simulink model "VirtualOscilloscope_stable"  (R2021b)
settings: Solver=VariableStepAuto  StartTime=0.0  StopTime=inf  MaxStep=0.001  RelTol=1e-3
PostLoadFcn:
  | % Resize the model window
  | set(0,"Units","pixels")
  | sSize = get(0,"screensize");
  | space =  sSize(4)*0.028;
  | set_param(gcs,'location',  [1,1,round(sSize(3)/2),sSize(4)-space]);
  | % Reset the zoom
  | set_param(gcs, 'ZoomFactor','FitSystem')
  | 
  | % Resize the windows
  | space = sSize(4)*0.032;
  | SAsize = ['[',num2str(round([(sSize(3)/2)+1,...
  |                     space,(sSize(3)/2)-1,sSize(4)/2-space*1.25])),']'];
  | DSOsize = ['[',num2str(round([(sSize(3)/2)+1,...
  |                   space/2+sSize(4)/2,(sSize(3)/2)-1,sSize(4)/2-1.25*space])),']'];
  | set_param([gcs,'/Signal Analyzer'],'WindowPosition',SAsize)
  | set_param([gcs,'/Oscilloscope'],'WindowPosition',DSOsize)
libraries: fl_lib x5, nesl_utility x3, simulink x2, ee_lib x1, dspxfrm3 x1
(part 1 of 2)
settings Model: Creator=Work  LastModifiedBy=Work

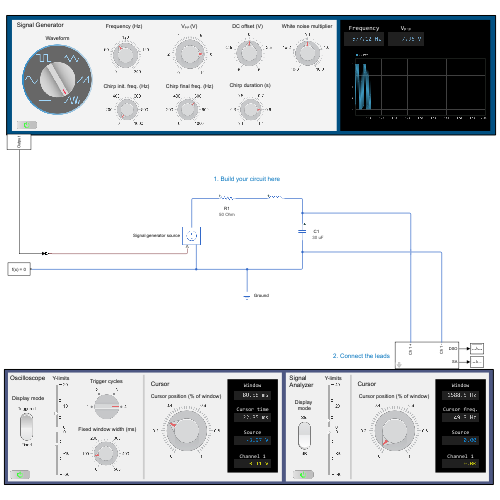
[thumbnail: Simulink's stored preview of the top-level diagram]
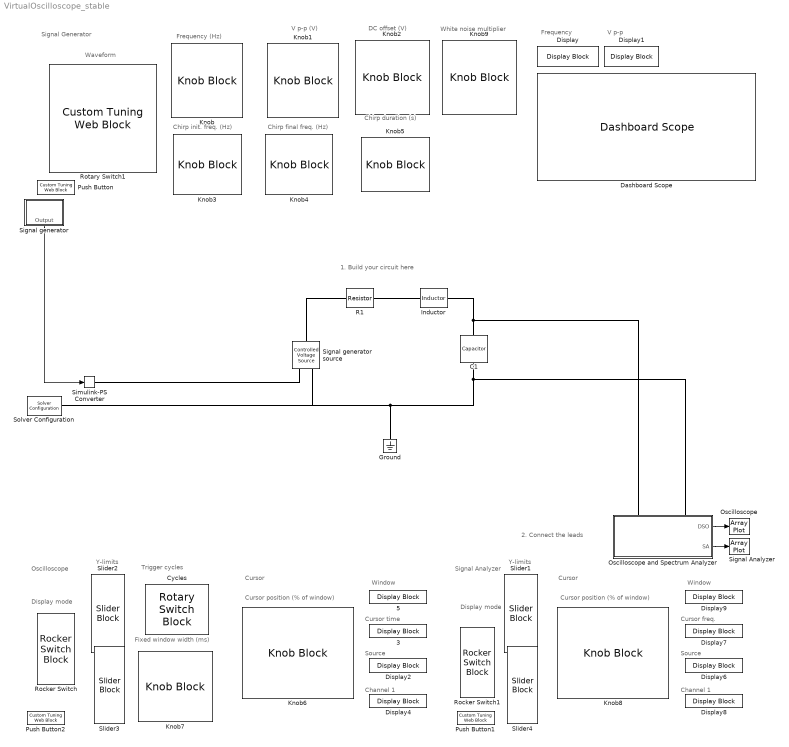
== system VirtualOscilloscope_stable ==
  note: 1. Build your circuit here
  note: Frequency (Hz)
  note: Waveform
  note: V p-p (V)
  note: Signal Generator
  note: Trigger cycles
  note: DC offset (V)
  note: Frequency
  note: V p-p
  note: Chirp init. freq. (Hz)
  note: Chirp final freq. (Hz)
  note: Source
  note: 2. Connect the leads
  note: Cursor position (% of window)
  note: Channel 1
  note: Cursor time
  note: Display mode
  note: Fixed window width (ms)
  note: Oscilloscope
  note: Window
  note: Cursor
  note: Window
  note: Cursor
  note: Channel 1
  note: Cursor position (% of window)
  note: Source
  note: Cursor freq.
  note: Chirp duration (s)
  note: Y-limits
  note: Display
      | mode
  note: Y-limits
  note: White noise multiplier
  note: Signal
      | Analyzer
  3 : DisplayBlock  LabelPosition=Hide  Format=Custom  Alignment=Right  Transparency=1  FormatString=%0.2f ms
  5 : DisplayBlock  LabelPosition=Hide  Format=Custom  Alignment=Right  Transparency=1  FormatString=%0.2f ms
  C1 : fl_lib/Electrical/Electrical Elements/Capacitor  c=30 uF  r=1e-6 Ohm  g=0 1/Ohm  i_specify=off  i_priority=None  i=0 A  i_nominal_specify=off  i_nominal_unit=A  i_nominal_value=1  v_specify=off  v_priority=None  v=0 V  v_nominal_specify=off  v_nominal_unit=V  v_nominal_value=1  vc_specify=off  vc_priority=High  vc=0 V  vc_nominal_specify=off  vc_nominal_unit=V  vc_nominal_value=1
      settings: AttributesFormatString=%<c> %<c_unit>
  Cycles : RotarySwitchBlock  LabelPosition=Hide
      settings: Values={{'1', '2', '3', '4'}, [1 2 3 4]}
  Dashboard Scope : DashboardScope  TimeSpan=0.20000000000000001  Ymin=-5  Ymax=5  ScaleAtStop=off
  Display : DisplayBlock  LabelPosition=Hide  Format=Custom  Alignment=Right  Transparency=1  FormatString=%0.2f Hz
  Display1 : DisplayBlock  LabelPosition=Hide  Format=Custom  Alignment=Right  Transparency=1  FormatString=%0.2f V
  Display2 : DisplayBlock  LabelPosition=Hide  Format=Custom  Alignment=Right  Transparency=1  FormatString=%0.2f V
  Display4 : DisplayBlock  LabelPosition=Hide  Format=Custom  Alignment=Right  Transparency=1  FormatString=%0.2f V
  Display6 : DisplayBlock  LabelPosition=Hide  Format=Custom  Alignment=Right  Transparency=1  FormatString=%0.2f
  Display7 : DisplayBlock  LabelPosition=Hide  Format=Custom  Alignment=Right  Transparency=1  FormatString=%0.1f Hz
  Display8 : DisplayBlock  LabelPosition=Hide  Format=Custom  Alignment=Right  Transparency=1  FormatString=%0.2f
  Display9 : DisplayBlock  LabelPosition=Hide  Format=Custom  Alignment=Right  Transparency=1  FormatString=%0.1f Hz
  Ground : fl_lib/Electrical/Electrical Elements/Electrical Reference
  Inductor : ee_lib/Passive/Inductor  l=0.1 H  L_tol=20  enable_L_tol=0  tol_distribution=1  nSigma=4  r=0 Ohm  g=1e-9 1/Ohm  enable_operating_limits=0  operating_limit_action=2  max_working_current=1 A  power_rating=1 W  enable_faults=0  fault_action=1  lambdaPercent=50  k_faulted=0.9999  turnsShort=0  openCct=0  groundShort=0  groundShortG=0 1/Ohm  tau_fault=1e-3 s  enable_temporal_fault=0  t_fault=1 s  enable_behavioral_fault=0  max_permissible_voltage=100 V  n_fail_on_voltage=1  max_permissible_current=1 A  t_fail_on_current=1 s  i_L_specify=off  i_L_priority=High  i_L=0 A  i_L_nominal_specify=off  i_L_nominal_unit=A  i_L_nominal_value=1
  Knob : KnobBlock  LabelPosition=Hide  ScaleMax=240  TickInterval=60
  Knob1 : KnobBlock  LabelPosition=Hide  ScaleMax=10  TickInterval=2
  Knob2 : KnobBlock  LabelPosition=Hide  ScaleMin=-5  ScaleMax=5  TickInterval=2.5
  Knob3 : KnobBlock  LabelPosition=Hide  ScaleMax=1000  TickInterval=200
  Knob4 : KnobBlock  LabelPosition=Hide  ScaleMax=1000  TickInterval=200
  Knob5 : KnobBlock  LabelPosition=Hide  ScaleMin=0.1  ScaleMax=1.1  TickInterval=0.2
  Knob6 : KnobBlock  LabelPosition=Hide  ScaleMax=1  TickInterval=0.2
  Knob7 : KnobBlock  LabelPosition=Hide  ScaleMax=500  TickInterval=100
  Knob8 : KnobBlock  LabelPosition=Hide  ScaleMax=1  TickInterval=0.2
  Knob9 : KnobBlock  LabelPosition=Hide  ScaleMin=1e-3  ScaleMax=10  ScaleType=Log
  Oscilloscope : ArrayPlot  WindowPosition=[1281.000000,743.000000,1279.000000,662.000000,]  Visible=on  PlotType=Line  AxesScaling=Manual  MaximizeAxes=off  YLimits=[-5.751633986928104,6.405228758169934]  ShowLegend=on
  Oscilloscope and Spectrum Analyzer : Subsystem  mask{Np=256, plot_dt=0.5e-5, refreshRate=100}
      mask prompts: Np "Sample points"; plot_dt "Sample time (s)"; refreshRate "Plot refresh rate (Hz)"
      settings: PortSchema="{\"entries\":[{\"content\":{\"sides\":[{\"content\":{\"connectorIds\":[\"LConn1\",\"LConn2\"]},\"type\":\"ConnectorPlacement.EquallySpacedRectSide\",\"uuid\":\"4f80a8c2-824d-4211-993f-82229c097a2c\"},{\"content\":{\"connectorIds\":[],\"side\":\"RIGHT\"},\"type\":\"ConnectorPlacement.EquallySpacedRectSide\",\"uuid\":\"5753fbaa-289b-4ec3-ae4c-c42164e19fcd\"},{\"content\":{\"connectorIds\":[\"Out1\",\"Out2\"],\"side\":\"TOP\"},\"type\":\"ConnectorPlacement.EquallySpacedRectSide\",\"uuid\":\"cde524b8-672e-4186-b31f-d28de61f9925\"}]},\"type\":\"ConnectorPlacement.EquallySpacedConnector\",\"uuid\":\"ab826d68-b3e0-4882-8d23-163848ab4439\"}],\"packageUris\":[\"http://schema.mathworks.com/mf0/Connector/R2020b\"],\"version\":\"1.0\"}"
  Push Button : CustomTuningWebBlock  LabelPosition=Hide  ShowInitialText=on  Configuration="{\"components\":[{\"name\":\"BackgroundImageComponent\",\"settings\":{\"image\":{\"size\":[0,0],\"src\":\"default\",\"srcOrientation\":\"horizontal\"},\"position\":[0,0,1,1],\"scaleMode\":\"0\"}},{\"name\":\"ButtonStateComponent\",\"settings\":{\"buttonType\":\"latch\",\"clickFcn\":\"\",\"latched\":true,\"offValue\":0,\"onValue\":1,\"position\":[0,0,1,1],\"pressDelay\":500,\"pressFcn\":\"\",\"repeatInterval\":0,\"states\":[{\"horizontalAlignment\":\"center\",\"image\":{\"position\":[0,0.07949909875723365,0.8410018024855327,1],\"size\":[0.8410018024855327,1],\"src\":\"data:image\\/png;base64,iVBORw0KGgoAAAANSUhEUgAAAk8AAAD+CAYAAAAjzuGXAAAACXBIWXMAAC4lAAAuJQH4pnvtAAAAGXRFWHRTb2Z0d2FyZQB3d3cuaW5rc2NhcGUub3Jnm+48GgAAIABJREFUeJzt3XlwHNmdH\\/jvyyqgTqCAKtwgSJDgfTXJNtmnRKK7R9LMyJJnvR7Je8xGeL3aXccqPLIVmlZPE85mt9QahRQay+GdjfGMZU9412PZO7cdY89oBTY9Gh3NJkV2N08QvAAQRxWAQhXqzrd\\/dAMiicxCHZmVWVXfTwRDYuXL937NArJ+9U4BeoSqqt5CoTAihBgGMCyEGBZC9EopI0KIiJQyAiAshBAA3FLKNlsDJiIiKpMQYgVAXkopAcSEEFEpZVQIEQXw ...(+19432 chars)\",\"srcOrientation\":\"Right\"},\"label\":{\"color\":[0.9176470588235294,0.9176470588235294,0.9176470588235294],\"icon\":{\"size\":[0,0],\"src\":\"default\",\"srcOrientation\":\"Right\"},\"iconPlacement\":\"left\",\"opacity\":1,\"show\":true,\"text\":{\"content\":\"\",\"font\":\"Helvetica\",\"fontSize\":42}},\"labelOffset\":[-0.019507668917408183,0.0018518518518518268],\"verticalAlignment\":\"middle\"},{\"horizontalAlignment\":\"center\",\"image\":{\"position\":[0,0.07949909875723365,0.8410018024855327,1],\"size\":[0.8410018024855327,1],\"src\":\"data:image\\/png;base64,iVBORw0KGgoAAAANSUhEUgAAAk8AAAD+CAYAAAAjzuGXAAAACXBIWXMAAC4lAAAuJQH4pnvtAAAAGXRFWHRTb2Z0d2FyZQB3d3cuaW5rc2NhcGUub3Jnm+48GgAAIABJREFUeJzt3Xl4HMd5J\\/5v9Qzmxn0SIAnwpkhLJCVRkkUdACVb8hErjje2c2zy28RxsnniTZx4bVkRuS1Kthw\\/9uPEOZx1fCTOL5eTOL5vWaBoS1F0ixIpkQQB3gCIe2Ywd9f+QQIEMN0z3T3dMwPi+9Ejm+h+u6pIipiXVW9XCdAiqqoGcrncBiFED4AeIUSPEKJdStkshGiWUjYDaBJCCABeKWVtRQdMRERkkRAiCiArpZQAJoQQ41LKcSHEOIBhAEML\\/j2pqm ...(+24250 chars)\",\"srcOrientation\":\"Right\"},\"label\":{\"color\":[0.9176470588235294,0.9176470588235294,0.9176470588235294],\"icon\":{\"size\":[0,0],\"src\":\"default\",\"srcOrientation\":\"Right\"},\"iconPlacement\":\"top\",\"opacity\":1,\"show\":true,\"text\":{\"content\":\"\",\"font\":\"Helvetica\",\"fontSize\":42}},\"labelOffset\":[-0.017384370015948947,0.002777777777777768],\"verticalAlignment\":\"middle\"},{\"horizontalAlignment\":\"center\",\"image\":{\"position\":[0,0.07949909875723365,0.8410018024855327,1],\"size\":[0.8410018024855327,1],\"src\":\"data:image\\/png;base64,iVBORw0KGgoAAAANSUhEUgAAAk8AAAD+CAYAAAAjzuGXAAAACXBIWXMAAC4lAAAuJQH4pnvtAAAAGXRFWHRTb2Z0d2FyZQB3d3cuaW5rc2NhcGUub3Jnm+48GgAAIABJREFUeJzt3Xl4HMd5J\\/5v9Qzmxn0SIAnwpkhLJCVRkkUdACVb8hErjje2c2zy28RxsnniTZx4bVkRuS1Kthw\\/9uPEOZx1fCTOL5eTOL5vWaBoS1F0ixIpkQQB3gCIe2Ywd9f+QQIEMN0z3T3dMwPi+9Ejm+h+u6pIipiXVW9XCdAiqqoGcrncBiFED4AeIUSPEKJdStkshGiWUjYDaBJCCABeKWVtRQdMRERkkRAiCiArpZQAJoQQ41LKcSHEOIBhAEML\\/j2pqm ...(+24250 chars)\",\"srcOrientation\":\"Right\"},\"label\":{\"color\":[0.9176470588235294,0.9176470588235294,0.9176470588235294],\"icon\":{\"size\":[0,0],\"src\":\"default\",\"srcOrientation\":\"Right\"},\"iconPlacement\":\"left\",\"opacity\":1,\"show\":true,\"text\":{\"content\":\"\",\"font\":\"Helvetica\",\"fontSize\":21}},\"labelOffset\":[0,0],\"verticalAlignment\":\"middle\"},{\"horizontalAlignment\":\"center\",\"image\":{\"position\":[0,0.07949909875723365,0.8410018024855327,1],\"size\":[0.8410018024855327,1],\"src\":\"data:image\\/png;base64,iVBORw0KGgoAAAANSUhEUgAAAk8AAAD+CAYAAAAjzuGXAAAACXBIWXMAAC4lAAAuJQH4pnvtAAAAGXRFWHRTb2Z0d2FyZQB3d3cuaW5rc2NhcGUub3Jnm+48GgAAIABJREFUeJzt3Xl4HMd5J\\/5v9Qzmxn0SIAnwpkhLJCVRkkUdACVb8hErjje2c2zy28RxsnniTZx4bVkRuS1Kthw\\/9uPEOZx1fCTOL5eTOL5vWaBoS1F0ixIpkQQB3gCIe2Ywd9f+QQIEMN0z3T3dMwPi+9Ejm+h+u6pIipiXVW9XCdAiqqoGcrncBiFED4AeIUSPEKJdStkshGiWUjYDaBJCCABeKWVtRQdMRERkkRAiCiArpZQAJoQQ41LKcSHEOIBhAEML\\/j2pqm ...(+24250 chars)\",\"srcOrientation\":\"Right\"},\"label\":{\"color\":[0.9176470588235294,0.9176470588235294,0.9176470588235294],\"icon\":{\"size\":[0,0],\"src\":\"default\",\"srcOrientation\":\"Right\"},\"iconPlacement\":\"left\",\"opacity\":1,\"show\":true,\"text\":{\"content\":\"\",\"font\":\"Helvetica\",\"fontSize\":21}},\"labelOffset\":[0.025,0],\"verticalAlignment\":\"middle\"}]}},{\"name\":\"ForegroundImageComponent\",\"settings\":{\"image\":{\"size\":[0,0],\"src\":\"default\",\"srcOrientation\":\"horizontal\"},\"isForeground\":1,\"position\":[0,0,1,1],\"scaleMode\":\"0\"}}],\"settings\":{\"BindingType\":\"param\",\"aspectRatio\":3.7777777777777777,\"backgroundColor\":[0,0,0,\"1\"],\"backgroundOffset\":0,\"backgroundOpacity\":1,\"fixedAspectRatio\":\"on\",\"foregroundColor\":[252,252,196],\"showBackgroundColor\":false,\"variant\":\"push\"},\"type\":\"Button\"}"
  Push Button1 : CustomTuningWebBlock  LabelPosition=Hide  ShowInitialText=on  Configuration="{\"components\":[{\"name\":\"BackgroundImageComponent\",\"settings\":{\"image\":{\"size\":[0,0],\"src\":\"default\",\"srcOrientation\":\"horizontal\"},\"position\":[0,0,1,1],\"scaleMode\":\"0\"}},{\"name\":\"ButtonStateComponent\",\"settings\":{\"buttonType\":\"latch\",\"clickFcn\":\"\",\"latched\":true,\"offValue\":0,\"onValue\":1,\"position\":[0,0,1,1],\"pressDelay\":500,\"pressFcn\":\"\",\"repeatInterval\":0,\"states\":[{\"horizontalAlignment\":\"center\",\"image\":{\"position\":[0,0.07949909875723365,0.8410018024855327,1],\"size\":[0.8410018024855327,1],\"src\":\"data:image\\/png;base64,iVBORw0KGgoAAAANSUhEUgAAAk8AAAD+CAYAAAAjzuGXAAAACXBIWXMAAC4lAAAuJQH4pnvtAAAAGXRFWHRTb2Z0d2FyZQB3d3cuaW5rc2NhcGUub3Jnm+48GgAAIABJREFUeJzt3XlwHNmdH\\/jvyyqgTqCAKtwgSJDgfTXJNtmnRKK7R9LMyJJnvR7Je8xGeL3aXccqPLIVmlZPE85mt9QahRQay+GdjfGMZU9412PZO7cdY89oBTY9Gh3NJkV2N08QvAAQRxWAQhXqzrd\\/dAMiicxCHZmVWVXfTwRDYuXL937NArJ+9U4BeoSqqt5CoTAihBgGMCyEGBZC9EopI0KIiJQyAiAshBAA3FLKNlsDJiIiKpMQYgVAXkopAcSEEFEpZVQIEQXw ...(+19432 chars)\",\"srcOrientation\":\"Right\"},\"label\":{\"color\":[0.9176470588235294,0.9176470588235294,0.9176470588235294],\"icon\":{\"size\":[0,0],\"src\":\"default\",\"srcOrientation\":\"Right\"},\"iconPlacement\":\"left\",\"opacity\":1,\"show\":true,\"text\":{\"content\":\"\",\"font\":\"Helvetica\",\"fontSize\":42}},\"labelOffset\":[-0.019507668917408183,0.0018518518518518268],\"verticalAlignment\":\"middle\"},{\"horizontalAlignment\":\"center\",\"image\":{\"position\":[0,0.07949909875723365,0.8410018024855327,1],\"size\":[0.8410018024855327,1],\"src\":\"data:image\\/png;base64,iVBORw0KGgoAAAANSUhEUgAAAk8AAAD+CAYAAAAjzuGXAAAACXBIWXMAAC4lAAAuJQH4pnvtAAAAGXRFWHRTb2Z0d2FyZQB3d3cuaW5rc2NhcGUub3Jnm+48GgAAIABJREFUeJzt3Xl4HMd5J\\/5v9Qzmxn0SIAnwpkhLJCVRkkUdACVb8hErjje2c2zy28RxsnniTZx4bVkRuS1Kthw\\/9uPEOZx1fCTOL5eTOL5vWaBoS1F0ixIpkQQB3gCIe2Ywd9f+QQIEMN0z3T3dMwPi+9Ejm+h+u6pIipiXVW9XCdAiqqoGcrncBiFED4AeIUSPEKJdStkshGiWUjYDaBJCCABeKWVtRQdMRERkkRAiCiArpZQAJoQQ41LKcSHEOIBhAEML\\/j2pqm ...(+24250 chars)\",\"srcOrientation\":\"Right\"},\"label\":{\"color\":[0.9176470588235294,0.9176470588235294,0.9176470588235294],\"icon\":{\"size\":[0,0],\"src\":\"default\",\"srcOrientation\":\"Right\"},\"iconPlacement\":\"top\",\"opacity\":1,\"show\":true,\"text\":{\"content\":\"\",\"font\":\"Helvetica\",\"fontSize\":42}},\"labelOffset\":[-0.017384370015948947,0.002777777777777768],\"verticalAlignment\":\"middle\"},{\"horizontalAlignment\":\"center\",\"image\":{\"position\":[0,0.07949909875723365,0.8410018024855327,1],\"size\":[0.8410018024855327,1],\"src\":\"data:image\\/png;base64,iVBORw0KGgoAAAANSUhEUgAAAk8AAAD+CAYAAAAjzuGXAAAACXBIWXMAAC4lAAAuJQH4pnvtAAAAGXRFWHRTb2Z0d2FyZQB3d3cuaW5rc2NhcGUub3Jnm+48GgAAIABJREFUeJzt3Xl4HMd5J\\/5v9Qzmxn0SIAnwpkhLJCVRkkUdACVb8hErjje2c2zy28RxsnniTZx4bVkRuS1Kthw\\/9uPEOZx1fCTOL5eTOL5vWaBoS1F0ixIpkQQB3gCIe2Ywd9f+QQIEMN0z3T3dMwPi+9Ejm+h+u6pIipiXVW9XCdAiqqoGcrncBiFED4AeIUSPEKJdStkshGiWUjYDaBJCCABeKWVtRQdMRERkkRAiCiArpZQAJoQQ41LKcSHEOIBhAEML\\/j2pqm ...(+24250 chars)\",\"srcOrientation\":\"Right\"},\"label\":{\"color\":[0.9176470588235294,0.9176470588235294,0.9176470588235294],\"icon\":{\"size\":[0,0],\"src\":\"default\",\"srcOrientation\":\"Right\"},\"iconPlacement\":\"left\",\"opacity\":1,\"show\":true,\"text\":{\"content\":\"\",\"font\":\"Helvetica\",\"fontSize\":21}},\"labelOffset\":[0,0],\"verticalAlignment\":\"middle\"},{\"horizontalAlignment\":\"center\",\"image\":{\"position\":[0,0.07949909875723365,0.8410018024855327,1],\"size\":[0.8410018024855327,1],\"src\":\"data:image\\/png;base64,iVBORw0KGgoAAAANSUhEUgAAAk8AAAD+CAYAAAAjzuGXAAAACXBIWXMAAC4lAAAuJQH4pnvtAAAAGXRFWHRTb2Z0d2FyZQB3d3cuaW5rc2NhcGUub3Jnm+48GgAAIABJREFUeJzt3Xl4HMd5J\\/5v9Qzmxn0SIAnwpkhLJCVRkkUdACVb8hErjje2c2zy28RxsnniTZx4bVkRuS1Kthw\\/9uPEOZx1fCTOL5eTOL5vWaBoS1F0ixIpkQQB3gCIe2Ywd9f+QQIEMN0z3T3dMwPi+9Ejm+h+u6pIipiXVW9XCdAiqqoGcrncBiFED4AeIUSPEKJdStkshGiWUjYDaBJCCABeKWVtRQdMRERkkRAiCiArpZQAJoQQ41LKcSHEOIBhAEML\\/j2pqm ...(+24250 chars)\",\"srcOrientation\":\"Right\"},\"label\":{\"color\":[0.9176470588235294,0.9176470588235294,0.9176470588235294],\"icon\":{\"size\":[0,0],\"src\":\"default\",\"srcOrientation\":\"Right\"},\"iconPlacement\":\"left\",\"opacity\":1,\"show\":true,\"text\":{\"content\":\"\",\"font\":\"Helvetica\",\"fontSize\":21}},\"labelOffset\":[0.025,0],\"verticalAlignment\":\"middle\"}]}},{\"name\":\"ForegroundImageComponent\",\"settings\":{\"image\":{\"size\":[0,0],\"src\":\"default\",\"srcOrientation\":\"horizontal\"},\"isForeground\":1,\"position\":[0,0,1,1],\"scaleMode\":\"0\"}}],\"settings\":{\"BindingType\":\"param\",\"aspectRatio\":3.7777777777777777,\"backgroundColor\":[0,0,0,\"1\"],\"backgroundOffset\":0,\"backgroundOpacity\":1,\"fixedAspectRatio\":\"on\",\"foregroundColor\":[252,252,196],\"showBackgroundColor\":false,\"variant\":\"push\"},\"type\":\"Button\"}"
  Push Button2 : CustomTuningWebBlock  LabelPosition=Hide  ShowInitialText=on  Configuration="{\"components\":[{\"name\":\"BackgroundImageComponent\",\"settings\":{\"image\":{\"size\":[0,0],\"src\":\"default\",\"srcOrientation\":\"horizontal\"},\"position\":[0,0,1,1],\"scaleMode\":\"0\"}},{\"name\":\"ButtonStateComponent\",\"settings\":{\"buttonType\":\"latch\",\"clickFcn\":\"\",\"latched\":true,\"offValue\":0,\"onValue\":1,\"position\":[0,0,1,1],\"pressDelay\":500,\"pressFcn\":\"\",\"repeatInterval\":0,\"states\":[{\"horizontalAlignment\":\"center\",\"image\":{\"position\":[0,0.07949909875723365,0.8410018024855327,1],\"size\":[0.8410018024855327,1],\"src\":\"data:image\\/png;base64,iVBORw0KGgoAAAANSUhEUgAAAk8AAAD+CAYAAAAjzuGXAAAACXBIWXMAAC4lAAAuJQH4pnvtAAAAGXRFWHRTb2Z0d2FyZQB3d3cuaW5rc2NhcGUub3Jnm+48GgAAIABJREFUeJzt3XlwHNmdH\\/jvyyqgTqCAKtwgSJDgfTXJNtmnRKK7R9LMyJJnvR7Je8xGeL3aXccqPLIVmlZPE85mt9QahRQay+GdjfGMZU9412PZO7cdY89oBTY9Gh3NJkV2N08QvAAQRxWAQhXqzrd\\/dAMiicxCHZmVWVXfTwRDYuXL937NArJ+9U4BeoSqqt5CoTAihBgGMCyEGBZC9EopI0KIiJQyAiAshBAA3FLKNlsDJiIiKpMQYgVAXkopAcSEEFEpZVQIEQXw ...(+19432 chars)\",\"srcOrientation\":\"Right\"},\"label\":{\"color\":[0.9176470588235294,0.9176470588235294,0.9176470588235294],\"icon\":{\"size\":[0,0],\"src\":\"default\",\"srcOrientation\":\"Right\"},\"iconPlacement\":\"left\",\"opacity\":1,\"show\":true,\"text\":{\"content\":\"\",\"font\":\"Helvetica\",\"fontSize\":42}},\"labelOffset\":[-0.019507668917408183,0.0018518518518518268],\"verticalAlignment\":\"middle\"},{\"horizontalAlignment\":\"center\",\"image\":{\"position\":[0,0.07949909875723365,0.8410018024855327,1],\"size\":[0.8410018024855327,1],\"src\":\"data:image\\/png;base64,iVBORw0KGgoAAAANSUhEUgAAAk8AAAD+CAYAAAAjzuGXAAAACXBIWXMAAC4lAAAuJQH4pnvtAAAAGXRFWHRTb2Z0d2FyZQB3d3cuaW5rc2NhcGUub3Jnm+48GgAAIABJREFUeJzt3Xl4HMd5J\\/5v9Qzmxn0SIAnwpkhLJCVRkkUdACVb8hErjje2c2zy28RxsnniTZx4bVkRuS1Kthw\\/9uPEOZx1fCTOL5eTOL5vWaBoS1F0ixIpkQQB3gCIe2Ywd9f+QQIEMN0z3T3dMwPi+9Ejm+h+u6pIipiXVW9XCdAiqqoGcrncBiFED4AeIUSPEKJdStkshGiWUjYDaBJCCABeKWVtRQdMRERkkRAiCiArpZQAJoQQ41LKcSHEOIBhAEML\\/j2pqm ...(+24250 chars)\",\"srcOrientation\":\"Right\"},\"label\":{\"color\":[0.9176470588235294,0.9176470588235294,0.9176470588235294],\"icon\":{\"size\":[0,0],\"src\":\"default\",\"srcOrientation\":\"Right\"},\"iconPlacement\":\"top\",\"opacity\":1,\"show\":true,\"text\":{\"content\":\"\",\"font\":\"Helvetica\",\"fontSize\":42}},\"labelOffset\":[-0.017384370015948947,0.002777777777777768],\"verticalAlignment\":\"middle\"},{\"horizontalAlignment\":\"center\",\"image\":{\"position\":[0,0.07949909875723365,0.8410018024855327,1],\"size\":[0.8410018024855327,1],\"src\":\"data:image\\/png;base64,iVBORw0KGgoAAAANSUhEUgAAAk8AAAD+CAYAAAAjzuGXAAAACXBIWXMAAC4lAAAuJQH4pnvtAAAAGXRFWHRTb2Z0d2FyZQB3d3cuaW5rc2NhcGUub3Jnm+48GgAAIABJREFUeJzt3Xl4HMd5J\\/5v9Qzmxn0SIAnwpkhLJCVRkkUdACVb8hErjje2c2zy28RxsnniTZx4bVkRuS1Kthw\\/9uPEOZx1fCTOL5eTOL5vWaBoS1F0ixIpkQQB3gCIe2Ywd9f+QQIEMN0z3T3dMwPi+9Ejm+h+u6pIipiXVW9XCdAiqqoGcrncBiFED4AeIUSPEKJdStkshGiWUjYDaBJCCABeKWVtRQdMRERkkRAiCiArpZQAJoQQ41LKcSHEOIBhAEML\\/j2pqm ...(+24250 chars)\",\"srcOrientation\":\"Right\"},\"label\":{\"color\":[0.9176470588235294,0.9176470588235294,0.9176470588235294],\"icon\":{\"size\":[0,0],\"src\":\"default\",\"srcOrientation\":\"Right\"},\"iconPlacement\":\"left\",\"opacity\":1,\"show\":true,\"text\":{\"content\":\"\",\"font\":\"Helvetica\",\"fontSize\":21}},\"labelOffset\":[0,0],\"verticalAlignment\":\"middle\"},{\"horizontalAlignment\":\"center\",\"image\":{\"position\":[0,0.07949909875723365,0.8410018024855327,1],\"size\":[0.8410018024855327,1],\"src\":\"data:image\\/png;base64,iVBORw0KGgoAAAANSUhEUgAAAk8AAAD+CAYAAAAjzuGXAAAACXBIWXMAAC4lAAAuJQH4pnvtAAAAGXRFWHRTb2Z0d2FyZQB3d3cuaW5rc2NhcGUub3Jnm+48GgAAIABJREFUeJzt3Xl4HMd5J\\/5v9Qzmxn0SIAnwpkhLJCVRkkUdACVb8hErjje2c2zy28RxsnniTZx4bVkRuS1Kthw\\/9uPEOZx1fCTOL5eTOL5vWaBoS1F0ixIpkQQB3gCIe2Ywd9f+QQIEMN0z3T3dMwPi+9Ejm+h+u6pIipiXVW9XCdAiqqoGcrncBiFED4AeIUSPEKJdStkshGiWUjYDaBJCCABeKWVtRQdMRERkkRAiCiArpZQAJoQQ41LKcSHEOIBhAEML\\/j2pqm ...(+24250 chars)\",\"srcOrientation\":\"Right\"},\"label\":{\"color\":[0.9176470588235294,0.9176470588235294,0.9176470588235294],\"icon\":{\"size\":[0,0],\"src\":\"default\",\"srcOrientation\":\"Right\"},\"iconPlacement\":\"left\",\"opacity\":1,\"show\":true,\"text\":{\"content\":\"\",\"font\":\"Helvetica\",\"fontSize\":21}},\"labelOffset\":[0.025,0],\"verticalAlignment\":\"middle\"}]}},{\"name\":\"ForegroundImageComponent\",\"settings\":{\"image\":{\"size\":[0,0],\"src\":\"default\",\"srcOrientation\":\"horizontal\"},\"isForeground\":1,\"position\":[0,0,1,1],\"scaleMode\":\"0\"}}],\"settings\":{\"BindingType\":\"param\",\"aspectRatio\":3.7777777777777777,\"backgroundColor\":[0,0,0,\"1\"],\"backgroundOffset\":0,\"backgroundOpacity\":1,\"fixedAspectRatio\":\"on\",\"foregroundColor\":[252,252,196],\"showBackgroundColor\":false,\"variant\":\"push\"},\"type\":\"Button\"}"
  R1 : fl_lib/Electrical/Electrical Elements/Resistor  R=50 Ohm  i_specify=off  i_priority=None  i=0 A  i_nominal_specify=off  i_nominal_unit=A  i_nominal_value=1  v_specify=off  v_priority=None  v=0 V  v_nominal_specify=off  v_nominal_unit=V  v_nominal_value=1
      settings: AttributesFormatString=%<R> %<R_unit>
  Rocker Switch : RockerSwitchBlock  LabelPosition=Hide
      settings: Values={{'Fixed', 'Triggered'}, [0 1]}
  Rocker Switch1 : RockerSwitchBlock  LabelPosition=Hide
      settings: Values={{'dB', 'Std'}, [0 1]}
  Rotary Switch1 : CustomTuningWebBlock  LabelPosition=Hide  ShowInitialText=on  Configuration="{\"components\":[{\"name\":\"RotarySwitchComponent\",\"settings\":{\"arcAngle\":300,\"arcAngleOffset\":120,\"handle\":{\"size\":[150,150],\"src\":\"data:image\\/svg+xml;base64,PHN2ZyBpZD0iTGF5ZXJfMSIgZGF0YS1uYW1lPSJMYXllciAxIiB4bWxucz0iaHR0cDovL3d3dy53My5vcmcvMjAwMC9zdmciIHhtbG5zOnhsaW5rPSJodHRwOi8vd3d3LnczLm9yZy8xOTk5L3hsaW5rIiB2aWV3Qm94PSIwIDAgMTIxIDEyMSI+PGRlZnM+PHN0eWxlPi5jbHMtMXtmaWxsOnVybCgjbGluZWFyLWdyYWRpZW50KTt9LmNscy0yLC5jbHMtM3tmaWxsOiNkMWQxZDE7fS5jbHMtM3tzdHJva2U6I2I3YjdiNztzdHJva2UtbWl0ZXJsaW1pdDoxMDtzdHJva2Utd2lkdGg6MC4yNXB4O30uY2xzLTR7ZmlsbDojZjMwMDAwO30uY2xzLTV7ZmlsbDojZjIxNzY3O308L3N0eWxlPjxsaW5lYXJHcmFkaWVudCBpZD0ibGluZWFyLWdyYWRpZW50IiB4MT0iNjAuNSIgeTE9IjEyMC41IiB4Mj0iNjAuNSIgeTI9IjAuNSIgZ3JhZGllbnRVbml0cz0idXNlclNwYWNlT25Vc2UiPjxzdG9wIG9mZnNldD0iMCIgc3RvcC1jb2xvcj0iI2QxZDFkMSIvPjxzdG9wIG9mZnNldD0iMC4xIiBzdG9wLWNvbG9yPSIjY2VjZWNlIi8+PHN0b3Agb2Zmc2V0PSIwLjE5IiBzdG9wLWNvbG9yPSIjYzNjM2MzIi8+PHN0b3Agb2Zmc2V0PSIwLjI4IiBzdG9wLWNvbG9yPSIjYjFiMWIxIi8+PHN0b3Agb2Zmc2V0PSIwLjM2IiBzdG9wLWNvbG9yPSIjOTg5ODk4Ii8+PHN0b3Agb2Zmc2V0PSIwLjQ0IiBzdG9wLWNvbG9yPSIjNzg3ODc4Ii8+PHN0b3Agb2Zmc2V0PSIwLjQ2IiBzdG9wLWNvbG9yPSIjNmI2YjZiIi8+PHN0b3Agb2Zmc2V0PSIwLjU0IiBzdG9wLWNvbG9yPSIjNmI2YjZiIi8+PHN0b3Agb2Zmc2V0PSIwLjU2IiBzdG9wLWNvbG9yPSIjNzY3Njc2Ii8+PHN0b3Agb2Zmc2V0PSIwLjY0IiBzdG9wLWNvbG9yPSIjOTc5Nzk3Ii8+PHN0b3Agb2Zmc2V0PSIwLjcyIiBzdG9wLWNvbG9yPSIjYjBiMGIwIi8+PHN0b3Agb2Zmc2V0PSIwLjgxIiBzdG9wLWNvbG9yPSIjYzNjM2MzIi8+PHN0b3Agb2Zmc2V0PSIwLjkiIHN0b3AtY29sb3I9IiNjZGNkY2QiLz48c3RvcCBvZmZzZXQ9IjEiIHN0b3AtY29sb3I9IiNkMWQxZDEiLz48L2xpbmVhckdyYWRpZW50PjwvZGVmcz48Y2lyY2xlIGNsYXNzPSJjbHMtMSIgY3g9IjYwLjUiIGN5PSI2MC41IiByPSI2MCIvPjxwYXRoIGNsYXNzPSJjbHMtMiIgZD0iTTYwLjUsMUE1OS41LDU5LjUsMCwxLDEsMSw2MC41LDU5LjU3LDU5LjU3LDAsMCwxLDYwLjUsMW0wLTFBNjAuNSw2MC41LDAsMSwwLDEyMSw2MC41LDYwLjUsNjAuNSwwLDAsMCw2MC41LDBaIi8+PHJlY3QgY2xhc3M9ImNscy0zIiB4PSIwLjUiIHk9IjUxLjUiIHdpZHRoPSIxMjAiIGhlaWdodD0iMTgiIHJ4PSIzLjA0Ii8+PHJlY3QgY2xhc3M9ImNscy00IiB4PSI1Ljc1IiB5PSI1OC43NSIgd2lkdGg9IjE2IiBoZWlnaHQ9IjMiLz48cGF0aCBjbGFzcz0iY2xzLTUiIGQ9Ik0yMS4yNSw1OS4yNXYyaC0xNXYtMmgxNW0xLTFoLTE3djRoMTd2LTRaIi8+PC9zdmc+\"},\"handleOffset\":[0,0],\"handleOrientation\":180,\"handlePosition\":[0,0,1,1],\"handleSize\":{\"height\":0.5,\"width\":0.5},\"labelRadius\":0.36,\"position\":[0,0,1,1],\"states\":[{\"Label\":{\"color\":[0,0,0],\"icon\":{\"size\":[1,1],\"src\":\"default\",\"srcOrientation\":\"Right\"},\"iconPlacement\":\"left\",\"opacity\":1,\"position\":[0,0],\"show\":true,\"text\":{\"content\":\"0\",\"fontSize\":14}},\"Value\":0},{\"Label\":{\"color\":[0,0,0,1],\"icon\":{\"size\":[0,0],\"src\":[],\"srcOrientation\":\"Right\"},\"iconPlacement\":\"left\",\"opacity\":1,\"position\":[0.35757211538461536,0.7603966346153846],\"show\":true,\"text\":{\"content\":\"1\",\"font\":\"Helvetica\",\"fontSize\":24}},\"Value\":1},{\"Label\":{\"color\":[0,0,0,1],\"icon\":{\"size\":[0,0],\"src\":[],\"srcOrientation\":\"Right\"},\"iconPlacement\":\"left\",\"opacity\":1,\"position\":[0.09603365384615385,0.46033653846153844],\"show\":true,\"text\":{\"content\":\"2\",\"font\":\"Helvetica\",\"fontSize\":24}},\"Value\":2},{\"Label\":{\"color\":[0,0,0,1],\"icon\":{\"size\":[0,0],\"src\":[],\"srcOrientation\":\"Right\"},\"iconPlacement\":\"left\",\"opacity\":1,\"position\":[0.36532451923076925,0.1180889423076923],\"show\":true,\"text\":{\"content\":\"3\",\"font\":\"Helvetica\",\"fontSize\":24}},\"Value\":3},{\"Label\":{\"color\":[0,0,0,1],\"icon\":{\"size\":[0,0],\"src\":[],\"srcOrientation\":\"Right\"},\"iconPlacement\":\"left\",\"opacity\":1,\"position\":[0.7191706730769231,0.19501201923076922],\"show\":true,\"text\":{\"content\":\"4\",\"font\":\"Helvetica\",\"fontSize\":24}},\"Value\":4},{\"Label\":{\"color\":[0,0,0],\"icon\":{\"size\":[1,1],\"src\":\"default\",\"srcOrientation\":\"Right\"},\"iconPlacement\":\"left\",\"opacity\":1,\"position\":[0,0],\"show\":true,\"text\":{\"content\":\"5\",\"fontSize\":14}},\"Value\":5}],\"tickRadius\":0.32}},{\"name\":\"BackgroundImageComponent\",\"settings\":{\"image\":{\"size\":[691,691],\"src\":\"data:image\\/png;base64,iVBORw0KGgoAAAANSUhEUgAAArMAAAKzCAYAAAAN54UbAAAACXBIWXMAAB7lAAAe5QGuvPLVAAAAGXRFWHRTb2Z0d2FyZQB3d3cuaW5rc2NhcGUub3Jnm+48GgAAIABJREFUeJzs3XlgVNX9NvDn3Fky2feFhAQSAkSCoLjigqAoCuJSFde27ra2te2vrVrtki7Wttra5a3VuuC+oLiiiCIBwg6CLGEPWYEsZN+TmXveP0IwQGaSzD2T2Z7PH5q5Z+6534Ew8+Tm3u8RICIKQjcsWBPqqLfGWDQRo2siRgIxUiBGA2IkRAyEjNagxQjALCGiIKRNQIQCMkIAFgkZIyAEgHAIWAFAfDO9GUDkscdC9I41A7Af91yBLgCtApAAGgTQLQVahESbEOiE ...(+67388 chars)\",\"srcOrientation\":\"Right\"},\"position\":[0,0,1,1],\"scaleMode\":\"0\"}},{\"name\":\"ForegroundImageComponent\",\"settings\":{\"image\":{\"size\":[0,0],\"src\":\"default\",\"srcOrientation\":[]},\"isForeground\":1,\"position\":[0,0,1,1],\"scaleMode\":\"0\"}}],\"settings\":{\"BindingType\":\"param\",\"backgroundColor\":[0,0,255,\"1\"],\"enumDataType\":\"\",\"fixedAspectRatio\":\"on\",\"image\":{\"size\":[150,150],\"src\":\"data:image\\/svg+xml;base64,PD94bWwgdmVyc2lvbj0iMS4wIiBlbmNvZGluZz0iVVRGLTgiIHN0YW5kYWxvbmU9Im5vIj8+CjwhLS0gR2VuZXJhdG9yOiBBZG9iZSBJbGx1c3RyYXRvciAxOS4yLjEsIFNWRyBFeHBvcnQgUGx1Zy1JbiAuIFNWRyBWZXJzaW9uOiA2LjAwIEJ1aWxkIDApICAtLT4KCjxzdmcKICAgeG1sbnM6ZGM9Imh0dHA6Ly9wdXJsLm9yZy9kYy9lbGVtZW50cy8xLjEvIgogICB4bWxuczpjYz0iaHR0cDovL2NyZWF0aXZlY29tbW9ucy5vcmcvbnMjIgogICB4bWxuczpyZGY9Imh0dHA6Ly93d3cudzMub3JnLzE5OTkvMDIvMjItcmRmLXN5bnRh ...(+9660 chars)\"},\"showBackgroundColor\":false,\"useEnumDataType\":false,\"variant\":\"rotarySwitch\"},\"type\":\"RotarySwitch\"}"
  Signal Analyzer : ArrayPlot  WindowPosition=[1281.000000,46.000000,1279.000000,662.000000,]  Visible=on  SampleIncrement=0.4200573221842449  PlotType=Line  AxesScaling=Manual  MaximizeAxes=off  YLimits=[-0.7741935483870961,5.935483870967742]  ShowLegend=on
  Signal generator : Subsystem
  Signal generator source : fl_lib/Electrical/Electrical Sources/Controlled Voltage Source
  Simulink-PS Converter : nesl_utility/Simulink-PS Converter  PhysicalDomain=network_engine_domain  SubClassName=ps_input  LeftPortType=input  RightPortType=output  PseudoPeriodic=off  Frequencies=[]  NoiseDistribution=none  NoiseParameters=[]  Unit=1  AffineConversion=off  FilteringAndDerivatives=provide  SimscapeFilterOrder=1  InputFilterTimeConstant=0.001  UdotUserProvided=0
      settings: SourceProductBaseCode=PW,SS
  Slider1 : SliderBlock  LabelPosition=Hide  ScaleMax=40  TickInterval=20
  Slider2 : SliderBlock  LabelPosition=Hide  ScaleMax=20  TickInterval=10
  Slider3 : SliderBlock  LabelPosition=Hide  ScaleMin=-20  ScaleMax=0  TickInterval=10
  Slider4 : SliderBlock  LabelPosition=Hide  ScaleMin=-40  ScaleMax=0  TickInterval=20
  Solver Configuration : nesl_utility/Solver Configuration  PhysicalDomain=network_engine_domain  SubClassName=solver  LeftPortType=input  RightPortType=generic  Tones=[]  Harmonics=[]  SimulateNoise=off  Profile=off  UseLocalSampling=off  EnableSwitchedLinearOptims=on  FrequencyDomain=off  UseCCode=off  RelTol=0.001  AbsTol=1e-06  MinStep=1e-09  ToWorkspace=off  RevertToSquareIcSolve=off  NumHomotopyIterations=100  PhasorMode=off  PhasorModeNumHarmonics=1  DoDC=off  ResidualTolerance=1e-09  UseLocalSolver=off  LocalSolverChoice=NE_BACKWARD_EULER_ADVANCER  LocalSolverSampleTime=0.001  DoFixedCost=off  MaxNonlinIter=3  MaxModeIter=2  ComputeImpulses=off  ImpulseIterations=2  LinearAlgebra=auto  EquationFormulation=NE_TIME_EF  DelaysMemoryBudget=1024  AutomaticFiltering=on  FilteringTimeConstant=0.001  PartitionStorageMethod=AS_NEEDED  PartitionMemoryBudget=1024  PartitionMethod=ROBUST
      settings: SourceProductBaseCode=PW,SS
  wires:
  Signal generator/1(Output) -> Simulink-PS Converter/1
  Oscilloscope and Spectrum Analyzer/1(DSO) -> Oscilloscope/1
  Oscilloscope and Spectrum Analyzer/2(SA) -> Signal Analyzer/1
  connections:
  Signal generator source/RConn2 -- Solver Configuration/RConn1 -- Ground/LConn1 -- Oscilloscope and Spectrum Analyzer/LConn1 -- C1/RConn1
  C1/LConn1 -- Oscilloscope and Spectrum Analyzer/LConn2 -- Inductor/RConn1
  Signal generator source/LConn1 -- R1/LConn1
  Simulink-PS Converter/RConn1 -- Signal generator source/RConn1
  Inductor/LConn1 -- R1/RConn1
